simulink library "rewardLibrary"  (R2022b)
settings: Solver=VariableStepAuto  StartTime=0.0  StopTime=10.0  RelTol=1e-3
values from neighbouring files (symbols this model uses):
  accel_vec = (-4:0.5:4)'    [setUpModel.m]
  Ts = 0.1    [setUpMPC.m]
  TsRL = Ts    [setUpRLEnv.m]
  vel_vec = 0:2:20    [setUpModel.m]
undefined symbols (not defined in the file or in its folder): A, B, C, curvature1, D, D_default, DiscIntNeverNeededParam, E, F, gradbp1, k_sigmoid, steer_lim, t_gap, v_set, x_colpen, y_colpen, Z_colpen
libraries: simulink x379, $bdroot x2, mpcadaslib x1
(part 9 of 9)

== system rewardLibrary/Obs // Reward 9-6/Path following ==
  v_err : Inport
  e1 : Inport  Port=2
  e2 : Inport  Port=3
  steer : Inport  Port=4
  accel : Inport  Port=5
  Constant : Constant  Commented=on  Value=0.5
  Exp{,1..4} (5 alike) : Math
  Gain1 : Gain  Gain=0.5
  Gain11 : Gain  Gain=-0.15
  Gain12 : Gain
  Gain2 : Gain  Gain=0.2
  Gain3 : Gain  Gain=0.1
  Gain4 : Gain  Gain=-0.9
  Gain5 : Gain  Gain=-10
  Gain6 : Gain  Gain=1.5
  Gain8 : Gain  Gain=-0.1
  Gain9 : Gain  Gain=-0.06
  Math Function2 : Math  Operator=square  SignedPower=on
  Square{1..4} (4 alike) : Math  Operator=square  SignedPower=on
  Sum1 : Sum  Inputs=++++++
  Unit Delay : UnitDelay  SampleTime=-1  HasFrameUpgradeWarning=on
  Unit Delay1 : UnitDelay  SampleTime=-1  HasFrameUpgradeWarning=on
  r_pf : Outport  VectorParamsAs1DForOutWhenUnconnected=off
  wires:
  Gain11/1 -> Exp/1
  Square4/1 -> Gain11/1
  Exp/1 -> Gain12/1
  v_err/1 -> Square4/1
  Sum1/1 -> r_pf/1
  accel/1 -> Unit Delay1/1
  Square2/1 -> Gain4/1
  steer/1 -> Unit Delay/1
  e1/1 -> Square1/1
  e2/1 -> Square2/1
  Unit Delay/1 -> Math Function2/1  "u_prev"
  Unit Delay1/1 -> Square3/1
  Square3/1 -> Gain8/1
  Math Function2/1 -> Gain5/1
  Square1/1 -> Gain9/1
  Gain8/1 -> Exp4/1
  Gain5/1 -> Exp3/1
  Gain4/1 -> Exp2/1
  Gain9/1 -> Exp1/1
  Exp1/1 -> Gain6/1
  Exp2/1 -> Gain1/1
  Exp3/1 -> Gain2/1
  Exp4/1 -> Gain3/1
  Gain3/1 -> Sum1/5
  Gain2/1 -> Sum1/4
  Gain1/1 -> Sum1/3
  Gain6/1 -> Sum1/2
  Gain12/1 -> Sum1/1
  Constant/1 -> Sum1/6

== system rewardLibrary/Obs // Reward 9-6/Subsystem ==
  v_ego : Inport
  v_ref : Inport  Port=2
  e1 : Inport  Port=3
  e2 : Inport  Port=4
  e1dot : Inport  Port=5
  e2dot : Inport  Port=6
  v_lead : Inport  Port=7
  xgap : Inport  Port=8
  ygap : Inport  Port=9
  Add : Sum  Inputs=+-
  Discrete-Time Integrator1 : DiscreteIntegrator  SampleTime=-1  ICPrevOutput=DiscIntNeverNeededParam  ICPrevScaledInput=DiscIntNeverNeededParam
  Discrete-Time Integrator2 : DiscreteIntegrator  SampleTime=-1  ICPrevOutput=DiscIntNeverNeededParam  ICPrevScaledInput=DiscIntNeverNeededParam
  Discrete-Time Integrator3 : DiscreteIntegrator  SampleTime=-1  ICPrevOutput=DiscIntNeverNeededParam  ICPrevScaledInput=DiscIntNeverNeededParam
  Lateral deviation : Scope
  Mux : Mux  Inputs=12
  obs : Outport  VectorParamsAs1DForOutWhenUnconnected=off
  v_err : Outport  Port=2  VectorParamsAs1DForOutWhenUnconnected=off
  wires:
  ygap/1 -> Mux/12
  xgap/1 -> Mux/11
  v_lead/1 -> Mux/10
  Add/1 -> v_err/1, Mux/2, Discrete-Time Integrator1/1
  Discrete-Time Integrator3/1 -> Mux/6  "integral_error"
  v_ego/1 -> Add/2, Mux/3
  e1/1 -> Lateral deviation/1, Mux/5, Discrete-Time Integrator2/1
  Discrete-Time Integrator1/1 -> Mux/1  "integral_error"
  e2/1 -> Mux/7, Discrete-Time Integrator3/1
  Discrete-Time Integrator2/1 -> Mux/4  "integral_error"
  Mux/1 -> obs/1
  e1dot/1 -> Mux/8
  e2dot/1 -> Mux/9
  v_ref/1 -> Add/1  "d_rel"

== system rewardLibrary/Obs // Reward 9-6/Subsystem2 ==
  v_ego : Inport
  e1 : Inport  Port=2
  e2 : Inport  Port=3
  xgap : Inport  Port=4
  collided : Inport  Port=5
  AND : Logic  IconShape=distinctive  AllPortsSameDT=off  OutDataTypeStr=boolean
  AND1 : Logic  IconShape=distinctive  AllPortsSameDT=off  OutDataTypeStr=boolean
  Abs : Abs  SaturateOnIntegerOverflow=off
  Abs1 : Abs  SaturateOnIntegerOverflow=off
  Compare To Constant : simulink/Logic and Bit Operations/Compare To Constant  relop=>  const=90  OutDataTypeStr=boolean
  Compare To Constant1 : simulink/Logic and Bit Operations/Compare To Constant  relop=>  const=0  OutDataTypeStr=boolean
  Constant : Constant
  Constant3 : Constant  Value=0
  Demux : Demux  Outputs=2
  Detect Rise Positive : simulink/Logic and Bit Operations/Detect Rise Positive  vinit=0  OutDataTypeStr=boolean
  Lateral deviation : simulink/Logic and Bit Operations/Compare To Constant  relop=>  const=8  OutDataTypeStr=boolean
  Logical Operator1 : Logic  Operator=OR  Inputs=3  AllPortsSameDT=off  OutDataTypeStr=boolean
  R2D : Gain  Gain=180/pi
  Relative yaw angle : simulink/Logic and Bit Operations/Compare To Constant  relop=>  const=40  OutDataTypeStr=boolean
  Switch : Switch  Criteria=u2 > Threshold  Threshold=90  SaturateOnIntegerOverflow=off  InputSameDT=off
  Terminator : Terminator
  Velocity : simulink/Logic and Bit Operations/Compare To Constant  relop=<  const=2  OutDataTypeStr=boolean
  Velocity1 : simulink/Logic and Bit Operations/Compare To Constant  relop=<  const=10  OutDataTypeStr=boolean
  fail : Outport  VectorParamsAs1DForOutWhenUnconnected=off
  failCollided : Outport  Port=2  VectorParamsAs1DForOutWhenUnconnected=off
  completeCourse : Outport  Port=3  VectorParamsAs1DForOutWhenUnconnected=off
  overtakeSuccess : Outport  Port=4  VectorParamsAs1DForOutWhenUnconnected=off
  wires:
  collided/1 -> failCollided/1
  AND1/1 -> overtakeSuccess/1
  Compare To Constant1/1 -> AND1/2
  xgap/1 -> Compare To Constant1/1
  Detect Rise Positive/1 -> AND1/1
  Compare To Constant/1 -> Detect Rise Positive/1
  Velocity/1 -> Logical Operator1/1  "tooSlow"
  Lateral deviation/1 -> Logical Operator1/2
  v_ego/1 -> Velocity1/1, Velocity/1
  Abs/1 -> Lateral deviation/1
  e1/1 -> Abs/1
  Velocity1/1 -> AND/1
  e2/1 -> Abs1/1
  Abs1/1 -> R2D/1
  R2D/1 -> Relative yaw angle/1
  Relative yaw angle/1 -> AND/2
  AND/1 -> Logical Operator1/3  "spinTurn"
  Switch/1 -> completeCourse/1
  Constant/1 -> Switch/1
  Constant3/1 -> Switch/3
  Logical Operator1/1 -> fail/1
  Demux/1 -> Terminator/1
  [pos2] -> Demux/1
  Demux/2 -> Switch/2, Compare To Constant/1  "y2"

== system rewardLibrary/Reward 0-0/Subsystem ==
  v_ego : Inport
  d_rel : Inport  Port=2
  v_lead : Inport  Port=3
  e1 : Inport  Port=4
  e2 : Inport  Port=5
  e1dot : Inport  Port=6
  e2dot : Inport  Port=7
  Discrete-Time Integrator1 : DiscreteIntegrator  SampleTime=-1  ICPrevOutput=DiscIntNeverNeededParam  ICPrevScaledInput=DiscIntNeverNeededParam
  Discrete-Time Integrator2 : DiscreteIntegrator  SampleTime=-1  ICPrevOutput=DiscIntNeverNeededParam  ICPrevScaledInput=DiscIntNeverNeededParam
  Discrete-Time Integrator3 : DiscreteIntegrator  SampleTime=-1  ICPrevOutput=DiscIntNeverNeededParam  ICPrevScaledInput=DiscIntNeverNeededParam
  Lateral deviation : Scope
  Mux : Mux  Inputs=9
  Subsystem1 : Subsystem
  Subsystem3 : Subsystem
  Subtract2 : Sum  Inputs=+-
  dist_comp : Scope  NumInputPorts=2
  obs : Outport  VectorParamsAs1DForOutWhenUnconnected=off
  v_err : Outport  Port=2  VectorParamsAs1DForOutWhenUnconnected=off
  wires:
  v_lead/1 -> Subsystem3/3(v_lead)
  Subsystem3/1(v_err) -> v_err/1, Mux/2, Discrete-Time Integrator1/1
  Discrete-Time Integrator3/1 -> Mux/6  "integral_error"
  v_ego/1 -> Mux/3, Subsystem3/2(v_ego), Subsystem1/1(v_ego)
  d_rel/1 -> dist_comp/2, Subtract2/2  "d_rel"
  e1/1 -> Lateral deviation/1, Mux/5, Discrete-Time Integrator2/1
  Subsystem1/1(safe_distance) -> dist_comp/1, Subtract2/1  "d_safe"
  Discrete-Time Integrator1/1 -> Mux/1  "integral_error"
  e2/1 -> Mux/7, Discrete-Time Integrator3/1
  Discrete-Time Integrator2/1 -> Mux/4  "integral_error"
  Mux/1 -> obs/1
  e1dot/1 -> Mux/8
  e2dot/1 -> Mux/9
  Subtract2/1 -> Subsystem3/1(d_err)

== system rewardLibrary/Reward 0-0/Subsystem1 ==
  u : Inport
  e1 : Inport  Port=2
  ev : Inport  Port=3
  a : Inport  Port=4
  Compare To Constant : simulink/Logic and Bit Operations/Compare To Constant  relop=<  const=1  OutDataTypeStr=boolean
  Compare To Constant1 : simulink/Logic and Bit Operations/Compare To Constant  relop=<  const=0.01  OutDataTypeStr=boolean
  Gain : Gain  Gain=100
  Gain2 : Gain  Gain=500
  Gain4 : Gain  Gain=1e-3
  Gain6 : Gain  Gain=100
  Gain7 : Gain  Gain=10
  Ht : Gain  Gain=2
  Math Function2 : Math  Operator=square  SignedPower=on
  Mt : Gain
  Square : Math  Operator=square  SignedPower=on
  Square2 : Math  Operator=square  SignedPower=on
  Square5 : Math  Operator=square  SignedPower=on
  Sum : Sum  Inputs=----
  Sum1 : Sum  Inputs=+++
  Unit Delay : UnitDelay  SampleTime=-1  HasFrameUpgradeWarning=on
  Unit Delay1 : UnitDelay  SampleTime=-1  HasFrameUpgradeWarning=on
  reward : Outport  VectorParamsAs1DForOutWhenUnconnected=off
  wires:
  e1/1 -> Square/1
  Gain/1 -> Sum/1
  Square/1 -> Compare To Constant1/1, Gain/1
  u/1 -> Unit Delay/1
  Square2/1 -> Gain2/1
  Unit Delay/1 -> Square2/1  "u_prev"
  a/1 -> Unit Delay1/1
  Unit Delay1/1 -> Math Function2/1  "a_prev"
  Square5/1 -> Compare To Constant/1, Gain7/1
  Math Function2/1 -> Gain6/1
  Gain7/1 -> Sum/3
  ev/1 -> Square5/1
  Gain6/1 -> Sum/4
  Gain2/1 -> Sum/2
  Sum1/1 -> reward/1
  Compare To Constant/1 -> Mt/1
  Mt/1 -> Sum1/3
  Compare To Constant1/1 -> Ht/1
  Ht/1 -> Sum1/1
  Sum/1 -> Gain4/1
  Gain4/1 -> Sum1/2

== system rewardLibrary/Reward 0-0/Subsystem2 ==
  d_rel : Inport
  v_ego : Inport  Port=2
  e1 : Inport  Port=3
  Abs : Abs  SaturateOnIntegerOverflow=off
  Lateral deviation : simulink/Logic and Bit Operations/Compare To Constant  relop=>  const=1  OutDataTypeStr=boolean
  Logical Operator : Logic  Operator=OR  Inputs=3  AllPortsSameDT=off  OutDataTypeStr=boolean
  Relative Distance : simulink/Logic and Bit Operations/Compare To Constant  relop=<  const=0  OutDataTypeStr=boolean
  Velocity : simulink/Logic and Bit Operations/Compare To Constant  relop=<  const=0.5  OutDataTypeStr=boolean
  isDone : Outport  VectorParamsAs1DForOutWhenUnconnected=off
  wires:
  Velocity/1 -> Logical Operator/2
  Relative Distance/1 -> Logical Operator/1
  d_rel/1 -> Relative Distance/1
  Logical Operator/1 -> isDone/1
  v_ego/1 -> Velocity/1
  Abs/1 -> Lateral deviation/1
  Lateral deviation/1 -> Logical Operator/3
  e1/1 -> Abs/1

== system rewardLibrary/Reward 1-1/Subsystem ==
  v_ego : Inport
  v_ref : Inport  Port=2
  e1 : Inport  Port=3
  e2 : Inport  Port=4
  e1dot : Inport  Port=5
  e2dot : Inport  Port=6
  Add : Sum  Inputs=+-
  Discrete-Time Integrator1 : DiscreteIntegrator  SampleTime=-1  ICPrevOutput=DiscIntNeverNeededParam  ICPrevScaledInput=DiscIntNeverNeededParam
  Discrete-Time Integrator2 : DiscreteIntegrator  SampleTime=-1  ICPrevOutput=DiscIntNeverNeededParam  ICPrevScaledInput=DiscIntNeverNeededParam
  Discrete-Time Integrator3 : DiscreteIntegrator  SampleTime=-1  ICPrevOutput=DiscIntNeverNeededParam  ICPrevScaledInput=DiscIntNeverNeededParam
  Lateral deviation : Scope
  Mux : Mux  Inputs=9
  obs : Outport  VectorParamsAs1DForOutWhenUnconnected=off
  v_err : Outport  Port=2  VectorParamsAs1DForOutWhenUnconnected=off
  wires:
  Add/1 -> v_err/1, Mux/2, Discrete-Time Integrator1/1
  Discrete-Time Integrator3/1 -> Mux/6  "integral_error"
  v_ego/1 -> Add/2, Mux/3
  e1/1 -> Lateral deviation/1, Mux/5, Discrete-Time Integrator2/1
  Discrete-Time Integrator1/1 -> Mux/1  "integral_error"
  e2/1 -> Mux/7, Discrete-Time Integrator3/1
  Discrete-Time Integrator2/1 -> Mux/4  "integral_error"
  Mux/1 -> obs/1
  e1dot/1 -> Mux/8
  e2dot/1 -> Mux/9
  v_ref/1 -> Add/1  "d_rel"

== system rewardLibrary/Reward 1-1/Subsystem1 ==
  steer : Inport
  e1 : Inport  Port=2
  v_err : Inport  Port=3
  accel : Inport  Port=4
  Compare To Constant1 : simulink/Logic and Bit Operations/Compare To Constant  relop=<  const=0.25  OutDataTypeStr=boolean
  Gain : Gain  Gain=100
  Gain1 : Gain  Gain=0
  Gain2 : Gain  Gain=200
  Gain3 : Gain  Gain=2
  Gain4 : Gain  Gain=1e-3
  Gain7 : Gain  Gain=10
  Square{,1..2,5} (4 alike) : Math  Operator=square  SignedPower=on
  Sum : Sum  Inputs=----
  Sum1 : Sum
  Unit Delay : UnitDelay  SampleTime=-1  HasFrameUpgradeWarning=on
  Unit Delay1 : UnitDelay  SampleTime=-1  HasFrameUpgradeWarning=on
  reward : Outport  VectorParamsAs1DForOutWhenUnconnected=off
  wires:
  e1/1 -> Square/1
  Gain/1 -> Sum/1
  Square/1 -> Compare To Constant1/1, Gain/1
  steer/1 -> Unit Delay/1
  Square2/1 -> Gain2/1
  Unit Delay/1 -> Square2/1
  Square5/1 -> Gain7/1
  Gain7/1 -> Sum/3
  v_err/1 -> Square5/1
  Gain2/1 -> Sum/2
  Sum1/1 -> reward/1
  Compare To Constant1/1 -> Gain3/1
  Gain3/1 -> Sum1/1
  Sum/1 -> Gain4/1
  Gain4/1 -> Sum1/2
  accel/1 -> Unit Delay1/1
  Unit Delay1/1 -> Square1/1
  Square1/1 -> Gain1/1
  Gain1/1 -> Sum/4

== system rewardLibrary/Reward 1-1/Subsystem2 ==
  v_ego : Inport
  e1 : Inport  Port=2
  Abs : Abs  SaturateOnIntegerOverflow=off
  Lateral deviation : simulink/Logic and Bit Operations/Compare To Constant  relop=>  const=8  OutDataTypeStr=boolean
  Logical Operator : Logic  Operator=OR  AllPortsSameDT=off  OutDataTypeStr=boolean
  Velocity : simulink/Logic and Bit Operations/Compare To Constant  relop=<  const=0.5  OutDataTypeStr=boolean
  isDone : Outport  VectorParamsAs1DForOutWhenUnconnected=off
  wires:
  Velocity/1 -> Logical Operator/1
  Logical Operator/1 -> isDone/1
  v_ego/1 -> Velocity/1
  Abs/1 -> Lateral deviation/1
  Lateral deviation/1 -> Logical Operator/2
  e1/1 -> Abs/1

== system rewardLibrary/Obs // Reward 3-3/Subsystem1/turn assist ==
  u_prev : Inport
  Abs : Abs  SaturateOnIntegerOverflow=off
  Constant : Constant  Value=steer_lim
  Constant1 : Constant  Value=0
  Gain10 : Gain  Gain=4444.4
  Square1 : Math  Operator=square  SignedPower=on
  Sum2 : Sum  Inputs=+-
  Switch1 : Switch  Criteria=u2 > Threshold  Threshold=0.02  SaturateOnIntegerOverflow=off  InputSameDT=off
  Out1 : Outport
  wires:
  Constant/1 -> Sum2/1
  Sum2/1 -> Square1/1
  Gain10/1 -> Switch1/1
  Switch1/1 -> Out1/1
  Abs/1 -> Switch1/2
  Constant1/1 -> Switch1/3
  u_prev/1 -> Sum2/2
  Square1/1 -> Gain10/1
  [curvature2] -> Abs/1

== system rewardLibrary/Obs // Reward 3-4/Subsystem1/turn assist ==
  u_prev : Inport
  Abs : Abs  SaturateOnIntegerOverflow=off
  Constant : Constant  Value=steer_lim
  Constant1 : Constant  Value=0
  Gain10 : Gain  Gain=4444.4
  Square1 : Math  Operator=square  SignedPower=on
  Sum2 : Sum  Inputs=+-
  Switch1 : Switch  Criteria=u2 > Threshold  Threshold=0.02  SaturateOnIntegerOverflow=off  InputSameDT=off
  Out1 : Outport
  wires:
  Constant/1 -> Sum2/1
  Sum2/1 -> Square1/1
  Gain10/1 -> Switch1/1
  Switch1/1 -> Out1/1
  Abs/1 -> Switch1/2
  Constant1/1 -> Switch1/3
  u_prev/1 -> Sum2/2
  Square1/1 -> Gain10/1
  [curvature2] -> Abs/1

== system rewardLibrary/Obs // Reward 3-5/Subsystem1/turn assist ==
  u_prev : Inport
  Abs : Abs  SaturateOnIntegerOverflow=off
  Constant : Constant  Value=steer_lim
  Constant1 : Constant  Value=0
  Gain10 : Gain  Gain=4444.4
  Square1 : Math  Operator=square  SignedPower=on
  Sum2 : Sum  Inputs=+-
  Switch1 : Switch  Criteria=u2 > Threshold  Threshold=0.02  SaturateOnIntegerOverflow=off  InputSameDT=off
  Out1 : Outport
  wires:
  Constant/1 -> Sum2/1
  Sum2/1 -> Square1/1
  Gain10/1 -> Switch1/1
  Switch1/1 -> Out1/1
  Abs/1 -> Switch1/2
  Constant1/1 -> Switch1/3
  u_prev/1 -> Sum2/2
  Square1/1 -> Gain10/1
  [curvature2] -> Abs/1

== system rewardLibrary/Obs // Reward 3-6/Subsystem1/turn assist ==
  u_prev : Inport
  Abs : Abs  SaturateOnIntegerOverflow=off
  Constant : Constant  Value=steer_lim
  Constant1 : Constant  Value=0
  Gain10 : Gain  Gain=4444.4
  Square1 : Math  Operator=square  SignedPower=on
  Sum2 : Sum  Inputs=+-
  Switch1 : Switch  Criteria=u2 > Threshold  Threshold=0.02  SaturateOnIntegerOverflow=off  InputSameDT=off
  Out1 : Outport
  wires:
  Constant/1 -> Sum2/1
  Sum2/1 -> Square1/1
  Gain10/1 -> Switch1/1
  Switch1/1 -> Out1/1
  Abs/1 -> Switch1/2
  Constant1/1 -> Switch1/3
  u_prev/1 -> Sum2/2
  Square1/1 -> Gain10/1
  [curvature2] -> Abs/1

== system rewardLibrary/Obs // Reward 4-1/Subsystem1/time reward ==
  Constant2 : Constant  Value=0
  Constant3 : Constant  Value=5
  Digital Clock : DigitalClock  SampleTime=Ts
  Switch2 : Switch  Criteria=u2 > Threshold  Threshold=10  SaturateOnIntegerOverflow=off  InputSameDT=off
  Out1 : Outport
  wires:
  Constant3/1 -> Switch2/1
  Switch2/1 -> Out1/1
  Digital Clock/1 -> Switch2/2
  Constant2/1 -> Switch2/3

== system rewardLibrary/Obs // Reward 4-1/Subsystem1/turn assist ==
  u_prev : Inport
  Abs : Abs  SaturateOnIntegerOverflow=off
  Constant : Constant  Value=steer_lim
  Constant1 : Constant  Value=0
  Gain10 : Gain  Gain=4444.4
  Square1 : Math  Operator=square  SignedPower=on
  Sum2 : Sum  Inputs=+-
  Switch1 : Switch  Criteria=u2 > Threshold  Threshold=0.02  SaturateOnIntegerOverflow=off  InputSameDT=off
  Out1 : Outport
  wires:
  Constant/1 -> Sum2/1
  Sum2/1 -> Square1/1
  Gain10/1 -> Switch1/1
  Switch1/1 -> Out1/1
  Abs/1 -> Switch1/2
  Constant1/1 -> Switch1/3
  u_prev/1 -> Sum2/2
  Square1/1 -> Gain10/1
  [curvature2] -> Abs/1

== system rewardLibrary/Obs // Reward 4-2/Subsystem1/time reward ==
  Constant2 : Constant  Value=0
  Constant3 : Constant  Value=5
  Digital Clock : DigitalClock  SampleTime=Ts
  Switch2 : Switch  Criteria=u2 > Threshold  Threshold=10  SaturateOnIntegerOverflow=off  InputSameDT=off
  Out1 : Outport
  wires:
  Constant3/1 -> Switch2/1
  Switch2/1 -> Out1/1
  Digital Clock/1 -> Switch2/2
  Constant2/1 -> Switch2/3

== system rewardLibrary/Obs // Reward 4-2/Subsystem1/turn assist ==
  u_prev : Inport
  Abs : Abs  SaturateOnIntegerOverflow=off
  Constant : Constant  Value=steer_lim
  Constant1 : Constant  Value=0
  Gain10 : Gain  Gain=4444.4
  Square1 : Math  Operator=square  SignedPower=on
  Sum2 : Sum  Inputs=+-
  Switch1 : Switch  Criteria=u2 > Threshold  Threshold=0.02  SaturateOnIntegerOverflow=off  InputSameDT=off
  Out1 : Outport
  wires:
  Constant/1 -> Sum2/1
  Sum2/1 -> Square1/1
  Gain10/1 -> Switch1/1
  Switch1/1 -> Out1/1
  Abs/1 -> Switch1/2
  Constant1/1 -> Switch1/3
  u_prev/1 -> Sum2/2
  Square1/1 -> Gain10/1
  [curvature2] -> Abs/1

== system rewardLibrary/Obs // Reward 6-2/Overtaking/Sigmoid ==
  x : Inport
  Add : Sum
  Constant : Constant
  Constant1 : Constant
  Divide : Product  Inputs=*/
  Exp : Math
  Gain1 : Gain  Gain=-0.25
  sigmoid : Outport
  wires:
  Divide/1 -> sigmoid/1
  Exp/1 -> Add/1
  x/1 -> Gain1/1
  Constant/1 -> Divide/1
  Gain1/1 -> Exp/1
  Constant1/1 -> Add/2
  Add/1 -> Divide/2

== system rewardLibrary/Obs // Reward 6-4/Subsystem1/expand this if needed ==
  In1 : Inport
  In2 : Inport  Port=2
  In3 : Inport  Port=3
  Add : Sum  Inputs=+-
  Constant : Constant
  Demux : Demux  Outputs=2
  Gain10 : Gain  Gain=0.1
  Gain7 : Gain  Gain=0.05
  Square5 : Math  Operator=square  SignedPower=on
  Switch : Switch  Criteria=u2 > Threshold  Threshold=-20  SaturateOnIntegerOverflow=off  InputSameDT=off
  Terminator : Terminator
  Out1 : Outport
  Out2 : Outport  Port=2
  wires:
  In3/1 -> Switch/3
  Switch/1 -> Out2/1
  Square5/1 -> Gain10/1
  Constant/1 -> Add/1
  In1/1 -> Square5/1
  Demux/1 -> Terminator/1
  [pos2] -> Demux/1
  Gain7/1 -> Out1/1
  Add/1 -> Gain7/1
  Gain10/1 -> Add/2
  In2/1 -> Switch/1
  Demux/2 -> Switch/2  "y2"

== system rewardLibrary/Obs // Reward 6-5/Subsystem1/expand this if needed ==
  In1 : Inport
  In2 : Inport  Port=2
  In3 : Inport  Port=3
  Add : Sum  Inputs=+-
  Constant : Constant
  Demux : Demux  Outputs=2
  Gain10 : Gain  Gain=0.1
  Gain7 : Gain  Gain=0.05
  Square5 : Math  Operator=square  SignedPower=on
  Switch : Switch  Criteria=u2 > Threshold  Threshold=-20  SaturateOnIntegerOverflow=off  InputSameDT=off
  Terminator : Terminator
  Out1 : Outport
  Out2 : Outport  Port=2
  wires:
  In3/1 -> Switch/3
  Switch/1 -> Out2/1
  Square5/1 -> Gain10/1
  Constant/1 -> Add/1
  In1/1 -> Square5/1
  Demux/1 -> Terminator/1
  [pos2] -> Demux/1
  Gain7/1 -> Out1/1
  Add/1 -> Gain7/1
  Gain10/1 -> Add/2
  In2/1 -> Switch/1
  Demux/2 -> Switch/2  "y2"

== system rewardLibrary/Obs // Reward 7-1/Overtaking/Sigmoid ==
  x : Inport
  Add : Sum
  Constant : Constant
  Constant1 : Constant
  Divide : Product  Inputs=*/
  Exp : Math
  Gain1 : Gain  Gain=-k_sigmoid
  sigmoid : Outport
  wires:
  Divide/1 -> sigmoid/1
  Exp/1 -> Add/1
  x/1 -> Gain1/1
  Constant/1 -> Divide/1
  Gain1/1 -> Exp/1
  Constant1/1 -> Add/2
  Add/1 -> Divide/2

== system rewardLibrary/Obs // Reward 7-2/Overtaking/Sigmoid ==
  x : Inport
  Add : Sum
  Constant : Constant
  Constant1 : Constant
  Divide : Product  Inputs=*/
  Exp : Math
  Gain1 : Gain  Gain=-k_sigmoid
  sigmoid : Outport
  wires:
  Divide/1 -> sigmoid/1
  Exp/1 -> Add/1
  x/1 -> Gain1/1
  Constant/1 -> Divide/1
  Gain1/1 -> Exp/1
  Constant1/1 -> Add/2
  Add/1 -> Divide/2

== system rewardLibrary/Obs // Reward 8-1/Overtaking/Sigmoid ==
  x : Inport
  Add : Sum
  Constant : Constant
  Constant1 : Constant
  Divide : Product  Inputs=*/
  Exp : Math
  Gain1 : Gain  Gain=-k_sigmoid
  sigmoid : Outport
  wires:
  Divide/1 -> sigmoid/1
  Exp/1 -> Add/1
  x/1 -> Gain1/1
  Constant/1 -> Divide/1
  Gain1/1 -> Exp/1
  Constant1/1 -> Add/2
  Add/1 -> Divide/2

== system rewardLibrary/Obs // Reward 8-10/Overtaking/Sigmoid ==
  x : Inport
  Add : Sum
  Constant : Constant
  Constant1 : Constant
  Divide : Product  Inputs=*/
  Exp : Math
  Gain1 : Gain  Gain=-0.25
  sigmoid : Outport
  wires:
  Add/1 -> Divide/2
  Constant1/1 -> Add/2
  Gain1/1 -> Exp/1
  Constant/1 -> Divide/1
  x/1 -> Gain1/1
  Exp/1 -> Add/1
  Divide/1 -> sigmoid/1

== system rewardLibrary/Obs // Reward 8-11/Overtaking/Sigmoid ==
  x : Inport
  Add : Sum
  Constant : Constant
  Constant1 : Constant
  Divide : Product  Inputs=*/
  Exp : Math
  Gain1 : Gain  Gain=-0.25
  sigmoid : Outport
  wires:
  Add/1 -> Divide/2
  Constant1/1 -> Add/2
  Gain1/1 -> Exp/1
  Constant/1 -> Divide/1
  x/1 -> Gain1/1
  Exp/1 -> Add/1
  Divide/1 -> sigmoid/1

== system rewardLibrary/Obs // Reward 8-12/Overtaking/Sigmoid ==
  x : Inport
  Add : Sum
  Constant : Constant
  Constant1 : Constant
  Divide : Product  Inputs=*/
  Exp : Math
  Gain1 : Gain  Gain=-0.25
  sigmoid : Outport
  wires:
  Add/1 -> Divide/2
  Constant1/1 -> Add/2
  Gain1/1 -> Exp/1
  Constant/1 -> Divide/1
  x/1 -> Gain1/1
  Exp/1 -> Add/1
  Divide/1 -> sigmoid/1

== system rewardLibrary/Obs // Reward 8-13/Overtaking/Sigmoid ==
  x : Inport
  Add : Sum
  Constant : Constant
  Constant1 : Constant
  Divide : Product  Inputs=*/
  Exp : Math
  Gain1 : Gain  Gain=-0.25
  sigmoid : Outport
  wires:
  Add/1 -> Divide/2
  Constant1/1 -> Add/2
  Gain1/1 -> Exp/1
  Constant/1 -> Divide/1
  x/1 -> Gain1/1
  Exp/1 -> Add/1
  Divide/1 -> sigmoid/1

== system rewardLibrary/Obs // Reward 8-14/Overtaking/lead ==
  x : Inport
  Add : Sum
  Constant : Constant
  Constant1 : Constant
  Divide : Product  Inputs=*/
  Exp : Math
  Gain1 : Gain  Gain=-0.6
  sigmoid : Outport
  wires:
  Add/1 -> Divide/2
  Constant1/1 -> Add/2
  Gain1/1 -> Exp/1
  Constant/1 -> Divide/1
  x/1 -> Gain1/1
  Exp/1 -> Add/1
  Divide/1 -> sigmoid/1

== system rewardLibrary/Obs // Reward 8-14/Overtaking/lead1 ==
  x : Inport
  Add : Sum
  Constant : Constant
  Constant1 : Constant
  Divide : Product  Inputs=*/
  Exp : Math
  Gain1 : Gain  Gain=-0.3
  sigmoid : Outport
  wires:
  Add/1 -> Divide/2
  Constant1/1 -> Add/2
  Gain1/1 -> Exp/1
  Constant/1 -> Divide/1
  x/1 -> Gain1/1
  Exp/1 -> Add/1
  Divide/1 -> sigmoid/1

== system rewardLibrary/Obs // Reward 8-15/Overtaking/lead ==
  x : Inport
  Add : Sum
  Constant : Constant
  Constant1 : Constant
  Divide : Product  Inputs=*/
  Exp : Math
  Gain1 : Gain  Gain=-0.6
  sigmoid : Outport
  wires:
  Add/1 -> Divide/2
  Constant1/1 -> Add/2
  Gain1/1 -> Exp/1
  Constant/1 -> Divide/1
  x/1 -> Gain1/1
  Exp/1 -> Add/1
  Divide/1 -> sigmoid/1

== system rewardLibrary/Obs // Reward 8-15/Overtaking/lead1 ==
  x : Inport
  Add : Sum
  Constant : Constant
  Constant1 : Constant
  Divide : Product  Inputs=*/
  Exp : Math
  Gain1 : Gain  Gain=-0.45
  sigmoid : Outport
  wires:
  Add/1 -> Divide/2
  Constant1/1 -> Add/2
  Gain1/1 -> Exp/1
  Constant/1 -> Divide/1
  x/1 -> Gain1/1
  Exp/1 -> Add/1
  Divide/1 -> sigmoid/1

== system rewardLibrary/Obs // Reward 8-16/Overtaking/lead ==
  x : Inport
  Add : Sum
  Constant : Constant
  Constant1 : Constant
  Divide : Product  Inputs=*/
  Exp : Math
  Gain1 : Gain  Gain=-0.6
  sigmoid : Outport
  wires:
  Add/1 -> Divide/2
  Constant1/1 -> Add/2
  Gain1/1 -> Exp/1
  Constant/1 -> Divide/1
  x/1 -> Gain1/1
  Exp/1 -> Add/1
  Divide/1 -> sigmoid/1

== system rewardLibrary/Obs // Reward 8-16/Overtaking/lead1 ==
  x : Inport
  Add : Sum
  Constant : Constant
  Constant1 : Constant
  Divide : Product  Inputs=*/
  Exp : Math
  Gain1 : Gain  Gain=-0.2
  sigmoid : Outport
  wires:
  Add/1 -> Divide/2
  Constant1/1 -> Add/2
  Gain1/1 -> Exp/1
  Constant/1 -> Divide/1
  x/1 -> Gain1/1
  Exp/1 -> Add/1
  Divide/1 -> sigmoid/1

== system rewardLibrary/Obs // Reward 8-2/Overtaking/Sigmoid ==
  x : Inport
  Add : Sum
  Constant : Constant
  Constant1 : Constant
  Divide : Product  Inputs=*/
  Exp : Math
  Gain1 : Gain  Gain=-k_sigmoid
  sigmoid : Outport
  wires:
  Divide/1 -> sigmoid/1
  Exp/1 -> Add/1
  x/1 -> Gain1/1
  Constant/1 -> Divide/1
  Gain1/1 -> Exp/1
  Constant1/1 -> Add/2
  Add/1 -> Divide/2

== system rewardLibrary/Obs // Reward 8-3/Overtaking/Sigmoid ==
  x : Inport
  Add : Sum
  Constant : Constant
  Constant1 : Constant
  Divide : Product  Inputs=*/
  Exp : Math
  Gain1 : Gain  Gain=-k_sigmoid
  sigmoid : Outport
  wires:
  Divide/1 -> sigmoid/1
  Exp/1 -> Add/1
  x/1 -> Gain1/1
  Constant/1 -> Divide/1
  Gain1/1 -> Exp/1
  Constant1/1 -> Add/2
  Add/1 -> Divide/2

== system rewardLibrary/Obs // Reward 8-4/Overtaking/Sigmoid ==
  x : Inport
  Add : Sum
  Constant : Constant
  Constant1 : Constant
  Divide : Product  Inputs=*/
  Exp : Math
  Gain1 : Gain  Gain=-k_sigmoid
  sigmoid : Outport
  wires:
  Divide/1 -> sigmoid/1
  Exp/1 -> Add/1
  x/1 -> Gain1/1
  Constant/1 -> Divide/1
  Gain1/1 -> Exp/1
  Constant1/1 -> Add/2
  Add/1 -> Divide/2

== system rewardLibrary/Obs // Reward 8-5/Overtaking/Sigmoid ==
  x : Inport
  Add : Sum
  Constant : Constant
  Constant1 : Constant
  Divide : Product  Inputs=*/
  Exp : Math
  Gain1 : Gain  Gain=-k_sigmoid
  sigmoid : Outport
  wires:
  Divide/1 -> sigmoid/1
  Exp/1 -> Add/1
  x/1 -> Gain1/1
  Constant/1 -> Divide/1
  Gain1/1 -> Exp/1
  Constant1/1 -> Add/2
  Add/1 -> Divide/2

== system rewardLibrary/Obs // Reward 8-7/Overtaking/Sigmoid ==
  x : Inport
  Add : Sum
  Constant : Constant
  Constant1 : Constant
  Divide : Product  Inputs=*/
  Exp : Math
  Gain1 : Gain  Gain=-0.25
  sigmoid : Outport
  wires:
  Divide/1 -> sigmoid/1
  Exp/1 -> Add/1
  x/1 -> Gain1/1
  Constant/1 -> Divide/1
  Gain1/1 -> Exp/1
  Constant1/1 -> Add/2
  Add/1 -> Divide/2

== system rewardLibrary/Obs // Reward 8-9/Overtaking/Sigmoid ==
  x : Inport
  Add : Sum
  Constant : Constant
  Constant1 : Constant
  Divide : Product  Inputs=*/
  Exp : Math
  Gain1 : Gain  Gain=-0.25
  sigmoid : Outport
  wires:
  Add/1 -> Divide/2
  Constant1/1 -> Add/2
  Gain1/1 -> Exp/1
  Constant/1 -> Divide/1
  x/1 -> Gain1/1
  Exp/1 -> Add/1
  Divide/1 -> sigmoid/1

== system rewardLibrary/Obs // Reward 9-3/Overtaking/Subsystem ==
  u : Inport
  In2 : Inport  Port=2
  In3 : Inport  Port=3
  In4 : Inport  Port=4
  u1 : Inport  Port=5
  AND : Logic  IconShape=distinctive  AllPortsSameDT=off  OutDataTypeStr=boolean
  Constant5 : Constant  Value=0
  G1 : Constant  Value=0.5
  Memory1 : Memory
  Overtake : simulink/Logic and Bit Operations/Compare To Constant  relop=>  const=0  OutDataTypeStr=boolean
  RHS : simulink/Logic and Bit Operations/Compare To Constant  relop=>  const=0  OutDataTypeStr=boolean
  RHS overtake? : Switch  Criteria=u2 > Threshold  SaturateOnIntegerOverflow=off  InputSameDT=off
  switch2 : Switch  Criteria=u2 > Threshold  SaturateOnIntegerOverflow=off  InputSameDT=off
  Out1 : Outport
  Out2 : Outport  Port=2
  wires:
  u1/1 -> RHS/1
  Overtake/1 -> AND/1
  switch2/1 -> Out1/1
  RHS overtake?/1 -> Out2/1
  u/1 -> Overtake/1
  Constant5/1 -> RHS overtake?/3
  G1/1 -> RHS overtake?/1
  In4/1 -> RHS overtake?/2
  RHS/1 -> AND/2
  In3/1 -> switch2/3
  In2/1 -> switch2/1
  AND/1 -> Memory1/1
  Memory1/1 -> switch2/2

== system rewardLibrary/Reward 0-0/Subsystem/Subsystem1 ==
  v_ego : Inport
  Default Spacing : Constant  Value=D_default  SampleTime=Ts
  Product : Product
  Sum2 : Sum
  Time Gap : Constant  Value=t_gap  SampleTime=Ts
  safe_distance : Outport  VectorParamsAs1DForOutWhenUnconnected=off
  wires:
  v_ego/1 -> Product/1
  Default Spacing/1 -> Sum2/1
  Time Gap/1 -> Product/2
  Product/1 -> Sum2/2
  Sum2/1 -> safe_distance/1

== system rewardLibrary/Reward 0-0/Subsystem/Subsystem3 ==
  d_err : Inport
  v_ego : Inport  Port=2
  v_lead : Inport  Port=3
  Constant : Constant  Value=v_set
  Min : MinMax  Inputs=2
  Sum1 : Sum  Inputs=+-
  Switch : Switch  Criteria=u2 > Threshold  SaturateOnIntegerOverflow=off  InputSameDT=off
  vel_comp : Scope  NumInputPorts=3
  v_err : Outport  VectorParamsAs1DForOutWhenUnconnected=off
  wires:
  v_lead/1 -> vel_comp/3, Min/1  "v_lead"
  Min/1 -> Switch/1
  Constant/1 -> Switch/3, vel_comp/2, Min/2  "v_set"
  d_err/1 -> Switch/2
  Switch/1 -> Sum1/1  "v_ref"
  v_ego/1 -> vel_comp/1, Sum1/2  "v_ego"
  Sum1/1 -> v_err/1
